simulink model "abs_project"  (R2020b)
settings: Solver=VariableStepAuto  StartTime=0.0  StopTime=10.0  RelTol=1e-3
PreLoadFcn:
  | l=5;
  | Kf=1;
  | PBmax=1500;
  | Rr=1.25;
  | TB=0.01;
  | ctrl=1;
  | g=32.18;
  | m=50;
  | v0=88;
model workspace (MAT data in the model file):
  I = 5
  Kf = 1
  PBmax = 1500
  Rr = 1.25
  TB = 0.01
  ctrl = 1
  g = 32.18
  m = 50
  mu = [0 0.4 0.8 0.97 1 0.98 0.96 0.94 0.92 0.9 0.88 0.855 0.83 0.81 0.79 0.77 0.75 0.73 0.72 0.71 0.7]
  slip = [0 0.05 0.1 0.15 0.2 0.25 0.3 0.35 0.4 0.45 0.5 0.55 0.6 0.65 0.7 0.75 0.8 0.85 0.9 0.95 1]
  v0 = 88
settings Model: Creator=com  LastModifiedBy=com
settings DebuggingCC: AlgebraicLoopMsg=none  ArtificialAlgebraicLoopMsg=none

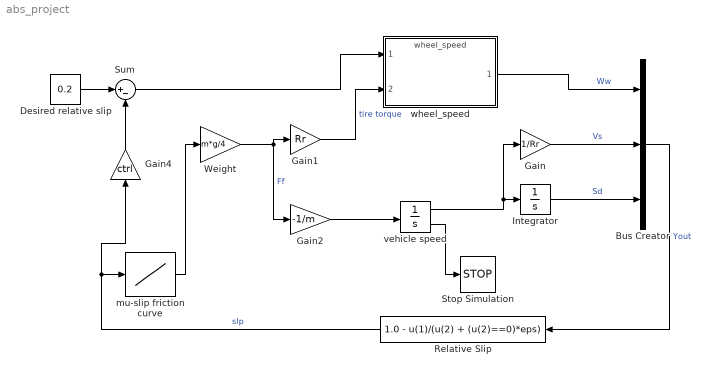
== system abs_project ==
  Bus Creator : BusCreator  Inputs=3
  Desired relative slip : Constant  Value=0.2
  Gain : Gain  Gain=1/Rr
  Gain1 : Gain  Gain=Rr
  Gain2 : Gain  Gain=-1/m
  Gain4 : Gain  Gain=ctrl
  Integrator : Integrator
  Relative Slip : Fcn  Expr=1.0 - u(1)/(u(2) + (u(2)==0)*eps)
  Stop Simulation : Stop
  Sum : Sum  Inputs=|+-
  Weight : Gain  Gain=m*g/4
  mu-slip friction curve : Lookup_n-D  NumberOfTableDimensions=1  BreakpointsForDimension1=slip  Table=mu  InternalRulePriority=Speed  RndMeth=Simplest  InputSameDT=on
  vehicle speed : Integrator  InitialCondition=v0  LimitOutput=on  UpperSaturationLimit=1000  LowerSaturationLimit=0  ShowSaturationPort=on
  wheel_speed : ModelReference  InitFcn=kf=1;  ModelNameDialog=wheel_speed  ModelReferenceVersion=1.11
  wires:
  Weight/1 -> Gain2/1, Gain1/1  "Ff"
  mu-slip friction curve/1 -> Weight/1
  Gain4/1 -> Sum/2
  Desired relative slip/1 -> Sum/1
  Gain2/1 -> vehicle speed/1
  vehicle speed/2 -> Stop Simulation/1
  vehicle speed/1 -> Gain/1, Integrator/1
  Integrator/1 -> Bus Creator/3  "Sd"
  Gain/1 -> Bus Creator/2  "Vs"
  wheel_speed/1 -> Bus Creator/1  "Ww"
  Gain1/1 -> wheel_speed/2  "tire torque"
  Bus Creator/1 -> Relative Slip/1  "Yout"
  Sum/1 -> wheel_speed/1
  Relative Slip/1 -> Gain4/1, mu-slip friction curve/1  "slp"
